simulink model "Sensors_and_actuators_ball_and_plate_2022b"  (R2022b)
settings: Solver=ode1  StartTime=0.0  StopTime=Inf  FixedStep=0.001  RelTol=1e-3
PostLoadFcn:
  | , if any(exist('dsrtsu_mdlpostloadfcn', 'file') ~= 0), dsrtsu_mdlpostloadfcn('Execute', bdroot); end,
InitFcn:
  | , if any(exist('rtifpga_mdlclblib', 'file') ~= 0), rtifpga_mdlclblib('Init', bdroot); end,
values from neighbouring files (symbols this model uses):
  a_y = ((0.1950)-(-0.1950))/(max_py-min_py)    [coordinate_transform.m]    (also in linearmap.m)
  b_x = -0.1950-(a_x*min_px)    [coordinate_transform.m]    (also in linearmap.m)
  b_y = -0.1950-(a_y*min_py)    [coordinate_transform.m]    (also in linearmap.m)
  center = cal1 + ((cal3-cal1)/2)    [coordinate_transform.m]    (also in linearmap.m)
libraries: rtiemclib x6, slpidlib x5, rtiethernetlib x3, rti1202lib_dac_class1 x3
(part 1 of 3)
Description:
  | Standard RTI1202 template.
  | Supported MATLAB version:  R2019b.
settings Model: Tag=RTI1202  DSRTSU_INTERNAL_RTI_VER=570  DSRTSU_INTERNAL_RTI_TYPE=rti1202  RTICANMMDATA=struct('GeneralSetupData',struct('modelroot','C:\Users\20203985\Documents\MATLAB\19_06_2023\simulink','generalsettings',struct('filesettings',struct('destfolder',struct('Name','RTICANMM_FILES','Check',1),'buildfolder',struct('Name','.','Check',1),'AbsDestfolder',struct('Name','C:\Users\20203985\Documents\MATLAB\19_06_2023\simulink\RTICANMM_FILES'),'AbsBuildfolder',struct('Name','C:\Users\20203985\Documents\MATLAB\19_06_2023\simulink'))),'options',struct('addpaths',1,'rmpaths',1,'addtrcexclusion',true,'cannavigator',struct('checkmonitoring',0),'show_usrtrc',0,'use_usrtrc',0),'advanced',struct('options',ones(1,100)),'MPSetup',{{}},'RTI',struct('Type','RTI1202','Ver','7.15','Date','02-Nov-2020'),'modelname','Sensors_and_actuators_ball_and_plate_2022b','block','Sensors_and_actuators_ball_and_plate_2022b'))  DSRTSU_INTERNAL_RTIFPGA=170  Creator=20201603  LastModifiedBy=20203985
settings SolverCC: AlgebraicLoopSolver=TrustRegion
settings DataIOCC: ReturnWorkspaceOutputs=off
settings OptimizationCC: BlockReduction=off  OptimizeBlockIOStorage=off  BufferReuse=off  GlobalBufferReuse=off  ExpressionFolding=off  LocalBlockOutputs=off  OptimizeDataStoreBuffers=off  BusAssignmentInplaceUpdate=off
settings DebuggingCC: ParameterOverflowMsg=none  UnconnectedInputMsg=warning  UnconnectedOutputMsg=warning  UnconnectedLineMsg=warning  PregeneratedLibrarySubsystemCodeDiagnostic=none  ArithmeticOperatorsInVariantConditions=warning
settings HardwareCC: ProdBitPerPointer=32  ProdBitPerSizeT=32  ProdBitPerPtrDiffT=32  ProdLargestAtomicInteger=Integer  ProdEndianess=BigEndian  ProdWordSize=32  ProdLongLongMode=on  ProdHWDeviceType=Custom Processor->Custom  TargetIntDivRoundTo=Zero  TargetEndianess=BigEndian  TargetHWDeviceType=Custom Processor->Custom
settings ModelReferenceCC: EnableRefExpFcnMdlSchedulingChecks=on  EnableParallelModelReferenceBuilds=on  ParallelModelReferenceMATLABWorkerInit=Load Top Model
settings SFSimCC: SimUseLocalCustomCode=off  MATLABDynamicMemAlloc=off  CustomCodeUndefinedFunction=UseInterfaceOnly
settings RTWCC: Description=dSPACE DS1202 Hardware Platform  SystemTargetFile=rti1202.tlc  MakeCommand=make_rti  TemplateMakefile=rti1202.tmf  RTWUseLocalCustomCode=off
settings CodeAppCC: StateflowObjectComments=on
settings STFCustomTargetCC: ParMdlRefBuildCompliant=on  SystemTargetFile=rti1202.tlc
settings GRTTargetCC: TargetLangStandard=C89/C90 (ANSI)  CompOptLevelCompliant=off  ConcurrentExecutionCompliant=off  CombineOutputUpdateFcns=off  MatFileLogging=off  CPPClassGenCompliant=off  UseToolchainInfoCompliant=off
settings ConfigComp: CovMetricSettings=dswe

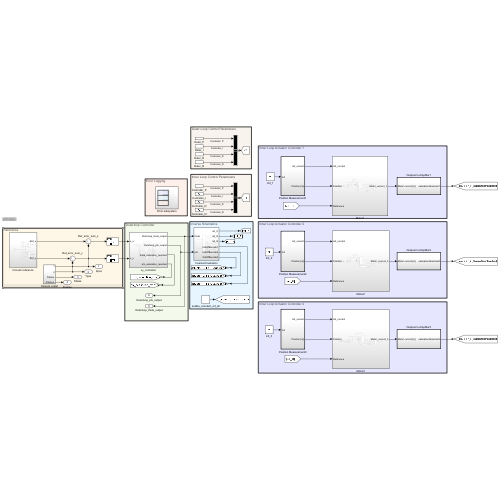
[thumbnail: Simulink's stored preview of the top-level diagram]
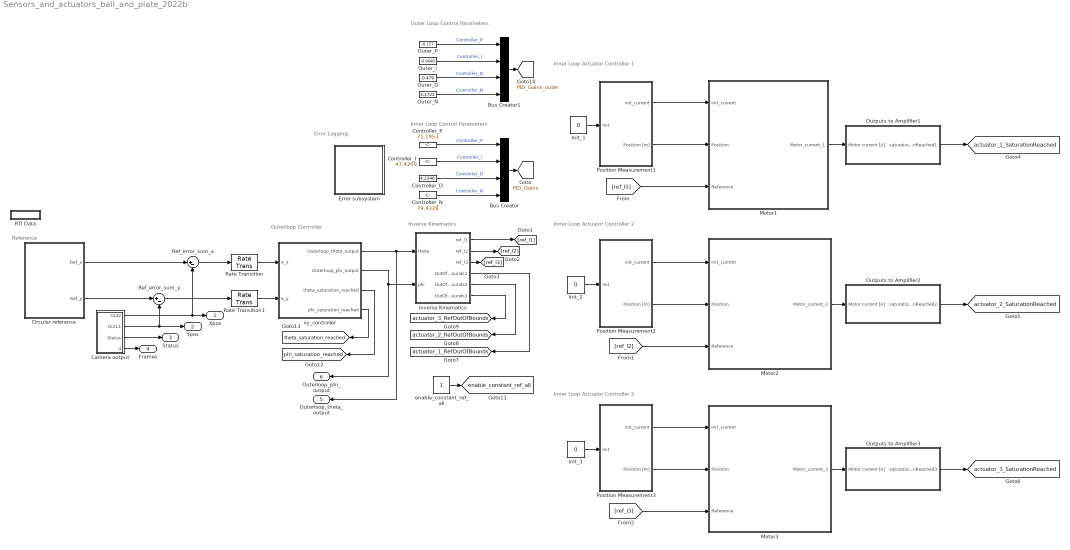
== system Sensors_and_actuators_ball_and_plate_2022b ==
  note: Inner Loop Control Parameters
  note: Error Logging
  note: Inverse Kinematics
  note: Inner Loop Actuator Controller 1
  note: Inner Loop Actuator Controller 2
  note: Inner Loop Actuator Controller 2
  note: Outerloop Controller
  note: Reference
  note: Outer Loop Control Parameters
  Bus Creator : BusCreator  Inputs=4
  Bus Creator1 : BusCreator  Inputs=4
  Camera output : Subsystem
  Circular reference : Subsystem
  Controller_D : Constant  Value=4.2346
  Controller_I : Constant  Value=47.4209
  Controller_N : Constant  Value=79.4328
  Controller_P : Constant  Value=71.1953
  Error subsystem : Subsystem
  Init_1 : Constant  Value=0
  Init_2 : Constant  Value=0
  Inverse Kinematics : Subsystem
  Motor1 : Subsystem
  Motor2 : Subsystem
  Motor3 : Subsystem
  Outer_D : Constant  Value=-0.479
  Outer_I : Constant  Value=-0.0648
  Outer_N : Constant  Value=3.1722
  Outer_P : Constant  Value=-0.157
  Outputs to Amplifier1 : Subsystem  TreatAsAtomicUnit=on
  Outputs to Amplifier2 : Subsystem  TreatAsAtomicUnit=on
  Outputs to Amplifier3 : Subsystem  TreatAsAtomicUnit=on
  Position Measurement1 : Subsystem  TreatAsAtomicUnit=on
  Position Measurement2 : Subsystem  TreatAsAtomicUnit=on
  Position Measurement3 : Subsystem  TreatAsAtomicUnit=on
  RTI Data : Subsystem  Tag=struct('RTIDataServer',struct('RTIDataServerVs','2','RTIModelDescription','struct(''main'',''Sensors_and_actuators_ball_and_plate_2022b'',''sub'','''',''isMp'',0)'))  LoadFcn="if exist('rtidc'), try,  rtidc('DataHostBlockClbLoad', gcbh); catch, disp(['Warning: ''LoadFcn'' for RTI Data block failed: ' lasterr]); end, end,"  mask(RTI_DATA_HOST){}
      mask help:
      | RTI Data Block.
      | This block is used by RTI to store internal model-dependent data.
      | Please keep this block on the root level of the model. Deleting this block will result in data loss.
      |
      | NEVER DELETE OR COPY THIS BLOCK!
      settings: CopyFcn="if exist('rtidc'), try,  rtidc('DataHostBlockClbCopy', gcbh); catch, disp(['Warning: ''CopyFcn'' for RTI Data block failed: ' lasterr]); end, end,"  DeleteFcn="if exist('rtidc'), try,  rtidc('DataHostBlockClbDelete', gcbh); catch, disp(['Warning: ''DeleteFcn'' for RTI Data block failed: ' lasterr]); end, end,"  ModelCloseFcn="if exist('rtidc'), try,  rtidc('DataHostBlockClbModelClose', gcbh); catch, disp(['Warning: ''ModelCloseFcn'' for RTI Data block failed: ' lasterr]); end, end,"  PreSaveFcn="if exist('rtidc'), try,  rtidc('DataHostBlockClbPreSave', gcbh); catch, disp(['Warning: ''PreSaveFcn'' for RTI Data block failed: ' lasterr]); end, end,"  PostSaveFcn="if exist('rtidc'), try,  rtidc('DataHostBlockClbPostSave', gcbh); catch, disp(['Warning: ''PostSaveFcn'' for RTI Data block failed: ' lasterr]); end, end,"  NameChangeFcn="if exist('rtidc'), try,  rtidc('DataHostBlockClbNameChange', gcbh); catch, disp(['Warning: ''NameChangeFcn'' for RTI Data block failed: ' lasterr]); end, end,"
      mask Help:
      | RTI Data Block.
      | This block is used by RTI to store internal model-dependent data.
      | Please keep this block on the root level of the model. Deleting this block will result in data loss.
      | 
      | NEVER DELETE OR COPY THIS BLOCK!
      mask Display:
      | text(0.5, 0.5, 'RTI Data', 'HorizontalAlignment', 'center');
      | plot([1 0]);
  Rate Transition : RateTransition  OutPortSampleTime=0.1
  Rate Transition1 : RateTransition  OutPortSampleTime=0.1
  Ref_error_sum_x : Sum  Inputs=|+-
  Ref_error_sum_y : Sum  Inputs=|+-
  enable_constant_ref_all : Constant
  init_3 : Constant  Value=0
  xy_controller : Subsystem
  "Xpos " : Outport
  "Ypos " : Outport  Port=2
  "Status " : Outport  Port=3
  "Frames " : Outport  Port=4
  Outerloop_theta_output : Outport  Port=5
  Outerloop_phi_output : Outport  Port=6
  tag scope: PID_Gains=global, PID_Gains_outer=global, actuator_1_RefOutOfBounds=global, actuator_1_SaturationReached=global, actuator_2_RefOutOfBounds=global, actuator_2_SaturationReached=global, actuator_3_RefOutOfBounds=global, actuator_3_SaturationReached=global, enable_constant_ref_all=global, phi_saturation_reached=global, theta_saturation_reached=global
  wires:
  Init_1/1 -> Position Measurement1/1(Init)
  init_3/1 -> Position Measurement3/1(Init)
  Controller_P/1 -> Bus Creator/1  "Controller_P"
  Controller_I/1 -> Bus Creator/2  "Controller_I"
  Controller_D/1 -> Bus Creator/3  "Controller_D"
  Controller_N/1 -> Bus Creator/4  "Controller_N"
  Position Measurement1/1(init_current) -> Motor1/1(Init_current)
  Position Measurement1/2(Position [m]) -> Motor1/2(Position)
  Motor1/1(Motor_current_1) -> Outputs to Amplifier1/1(Motor current [A])
  Position Measurement2/1(init_current) -> Motor2/1(Init_current)
  Position Measurement2/2(Position [m]) -> Motor2/2(Position)
  Motor2/1(Motor_current_2) -> Outputs to Amplifier2/1(Motor current [A])
  Position Measurement3/1(init_current) -> Motor3/1(Init_current)
  Position Measurement3/2(Position [m]) -> Motor3/2(Position)
  Motor3/1(Motor_current_3) -> Outputs to Amplifier3/1(Motor current [A])
  Circular reference/1(Ref_x) -> Ref_error_sum_x/1
  Circular reference/2(Ref_y) -> Ref_error_sum_y/1
  Camera output/1(Out2) -> "Xpos "/1, Ref_error_sum_x/2
  Camera output/2(Out11) -> "Ypos "/1, Ref_error_sum_y/2
  Camera output/3("Status ") -> "Status "/1
  Camera output/4("Frames ") -> "Frames "/1
  Ref_error_sum_x/1 -> Rate Transition/1
  Ref_error_sum_y/1 -> Rate Transition1/1
  Init_2/1 -> Position Measurement2/1(Init)
  Inverse Kinematics/2(ref_l2) -> [ref_l2]
  Inverse Kinematics/3(ref_l3) -> [ref_l3]
  Inverse Kinematics/1(ref_l1) -> [ref_l1]
  [ref_l1] -> Motor1/3(Reference)
  [ref_l2] -> Motor2/3(Reference)
  [ref_l3] -> Motor3/3(Reference)
  xy_controller/1(Outerloop_theta_output) -> Outerloop_theta_output/1, Inverse Kinematics/1(theta)
  xy_controller/2(Outerloop_phi_output) -> Outerloop_phi_output/1, Inverse Kinematics/2(phi)
  Bus Creator/1 -> [PID_Gains]
  Inverse Kinematics/4(OutOfBounds1) -> [actuator_1_RefOutOfBounds]
  Inverse Kinematics/5(OutOfBounds2) -> [actuator_2_RefOutOfBounds]
  Inverse Kinematics/6(OutOfBounds3) -> [actuator_3_RefOutOfBounds]
  Outputs to Amplifier1/1(saturationReached1) -> [actuator_1_SaturationReached]
  Outputs to Amplifier2/1(saturationReached2) -> [actuator_2_SaturationReached]
  Outputs to Amplifier3/1(saturationReached3) -> [actuator_3_SaturationReached]
  Outer_N/1 -> Bus Creator1/4  "Controller_N"
  Bus Creator1/1 -> [PID_Gains_outer]
  Outer_D/1 -> Bus Creator1/3  "Controller_D"
  Outer_P/1 -> Bus Creator1/1  "Controller_P"
  Outer_I/1 -> Bus Creator1/2  "Controller_I"
  enable_constant_ref_all/1 -> [enable_constant_ref_all]
  xy_controller/4(phi_saturation_reached) -> [theta_saturation_reached]
  xy_controller/3(theta_saturation_reached) -> [phi_saturation_reached]
  Rate Transition/1 -> xy_controller/1(e_x)
  Rate Transition1/1 -> xy_controller/2(e_y)

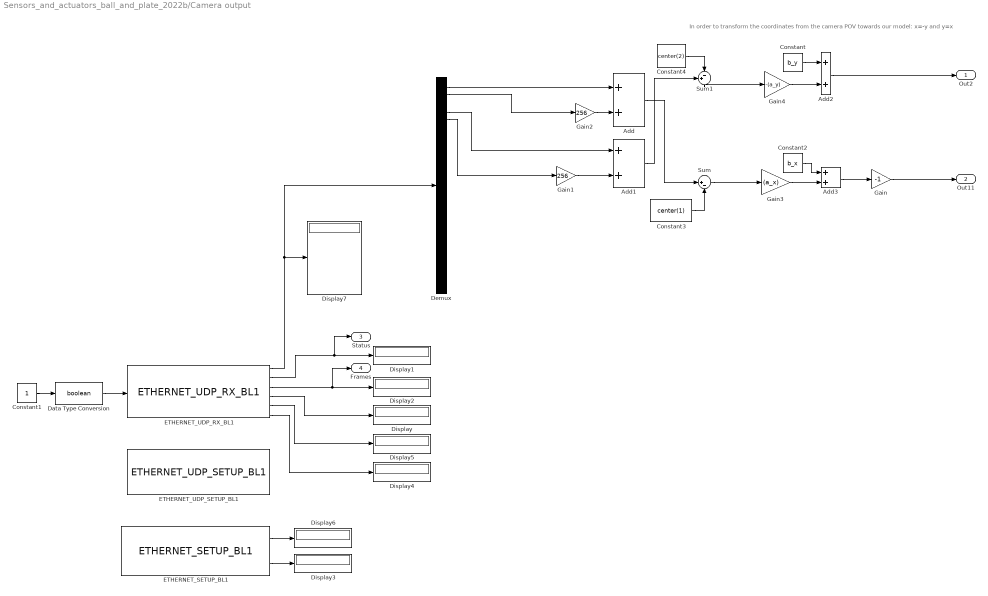
== system Sensors_and_actuators_ball_and_plate_2022b/Camera output ==
  note: In order to transform the coordinates from the camera POV towards our model: x=-y and y=x
  Add : Sum  AccumDataTypeStr=uint16
  Add1 : Sum
  Add2 : Sum
  Add3 : Sum
  Constant : Constant  Value=b_y
  Constant1 : Constant
  Constant2 : Constant  Value=b_x
  Constant3 : Constant  Value=center(1)
  Constant4 : Constant  Value=center(2)
  Data Type Conversion : DataTypeConversion  OutDataTypeStr=boolean  SaturateOnIntegerOverflow=off  RndMeth=Floor
  Demux : Demux  Outputs=32
  Display{,1..7} (8 alike) : Display
      Display7 settings: Format=decimal (Stored Integer)
  ETHERNET_SETUP_BL1 : rtiethernetlib/ETHERNET_SETUP_BL1  DSProperties=struct('RTI',struct('Version',uint32(2),'BlockType',struct('isSLSource',uint8(0),'isSLSink',uint8(0),'isHWSource',uint8(0),'isHWSink',uint8(0),'isSetup',uint8(1),'isInline',uint8(1),'isNonInline',uint8(0),'isInterrupt',uint8(0),'isChannelwise',uint8(0)),'IOBoardType','DSETHERNET','UnitType','ETHERNET','Identifier','SETUP','DialogType','ML','BlockSet','RTIETHERNET','SlaveProcessor','NONE'))  RTIBlockInterface=struct('OutputPortsWidth',int32([3 1 1 4]),'OutputPortsActive',[1 0 0 1],'OutputPortsName',{{['Link Status'],['Watchdog Status'],['DHCP Status'],['Local IP']}},'OutputPortsDataType',{{'SS_UINT32','SS_UINT32','SS_UINT32','SS_UINT8'}},'InitLevel',3,'IconTransparency','on','BlockDisplay',{{['Ethernet Setup\n\nLocal IP: 192.168.141.7'],'left'}},'DialogFcn','rtiethernetsetupgui','BlockName',struct('Token',{{'ETHERNET_SETUP_BL1'}}))  RTIBlockParameters=struct('DHCPserverMode',{{0,'OFF',[0 1]}},'LocalIpNum1',{{'192','OFF',[0 255]}},'LocalIpNum2',{{'168','OFF',[0 255]}},'LocalIpNum3',{{'141','OFF',[0 255]}},'LocalIpNum4',{{'7','OFF',[0 255]}},'SubnetMaskNum1',{{'255','OFF',[0 255]}},'SubnetMaskNum2',{{'255','OFF',[0 255]}},'SubnetMaskNum3',{{'255','OFF',[0 255]}},'SubnetMaskNum4',{{'0','OFF',[0 255]}},'GatewayNum1',{{'0','OFF',[0 255]}},'GatewayNum2',{{'0','OFF',[0 255]}},'GatewayNum3',{{'0','OFF',[0 255]}},'GatewayNum4',{{'0','OFF',[0 255]}},'LinkStatusOutPortMode',{{1,'OFF',[0 1]}},'NumOfEthConnectors',{{3,'ON',[1 16]}},'WatchdogStatusOutPortMode',{{0,'OFF',[0 1]}},'LocalIpOutPortMode',{{1,'OFF',[0 1]}},'IpAndSubmaskCheck',{{int32(1),'OFF',[0 1]}},'TLCFileName',{{'rtiethernetsetup','OFF',[]}})  RTISFcnParameters=struct('DHCPserverMode','int32','LocalIpNum1','uint8','LocalIpNum2','uint8','LocalIpNum3','uint8','LocalIpNum4','uint8','SubnetMaskNum1','uint8','SubnetMaskNum2','uint8','SubnetMaskNum3','uint8','SubnetMaskNum4','uint8','GatewayNum1','uint8','GatewayNum2','uint8','GatewayNum3','uint8','GatewayNum4','uint8','LinkStatusOutPortMode','int32','NumOfEthConnectors','int32','WatchdogStatusOutPortMode','int32','LocalIpOutPortMode','int32','TLCFileName','char')  RTIBlockParaDefault=struct('DHCPserverMode',0,'LocalIpNum1',192,'LocalIpNum2',168,'LocalIpNum3',140,'LocalIpNum4',6,'SubnetMaskNum1',255,'SubnetMaskNum2',255,'SubnetMaskNum3',255,'SubnetMaskNum4',0,'GatewayNum1',0,'GatewayNum2',0,'GatewayNum3',0,'GatewayNum4',0,'LinkStatusOutPortMode',1,'NumOfEthConnectors',3,'WatchdogStatusOutPortMode',0,'LocalIpOutPortMode',0,'IpAndSubmaskCheck',1,'TLCFileName','rtiethernetsetup')
      settings: SourceProductName=dSPACE RTI Ethernet Blockset
  ETHERNET_UDP_RX_BL1 : rtiethernetlib/ETHERNET_UDP_RX_BL1  DSProperties=struct('RTI',struct('Version',uint32(1),'BlockType',struct('isSLSource',uint8(1),'isSLSink',uint8(1),'isHWSource',uint8(0),'isHWSink',uint8(1),'isSetup',uint8(0),'isInline',uint8(1),'isNonInline',uint8(0),'isInterrupt',uint8(0),'isChannelwise',uint8(0)),'IOBoardType','DSETHERNET','UnitType','UDP','Identifier','RXUDP','DialogType','ML','BlockSet','RTIETHERNET','SlaveProcessor','NONE'))  RTIBlockInterface=struct('OutputPortsWidth',int32([32 1 1 1 4 1]),'OutputPortsActive',[1 1 1 1 1 1],'OutputPortsName',{{'Data','Status',['Received Frames'],['Received Bytes'],['Remote IP'],['Remote Port']}},'OutputPortsDataType',{{'SS_UINT8','SS_UINT32','SS_DOUBLE','SS_UINT32','SS_UINT8','SS_UINT16'}},'InputPortsWidth',int32(1),'InputPortsActive',1,'InputPortsName',{{'Enable'}},'InputPortsDataType',{{'SS_BOOLEAN'}},'RWork',{{{'RECEIVED_FRAMES',uint32(1)}}},'InitLevel',3,'IconTransparency','on','BlockDisplay',{{['Ethernet UDP/IP\nRX\n\nSocket ID: 0'],'center'}},'DialogFcn','rtiethernetrxudpgui','BlockName',struct('Token',{{'ETHERNET_UDP_RX_BL1'}}))  RTIBlockParameters=struct('SocketIdIndex',{{2,'OFF',[1 2]}},'SocketId',{{0,'OFF',[-1 inf]}},'RemoteIp',{{['<NOT AVAILABLE>'],'OFF',[]}},'RemotePort',{{['<NOT AVAILABLE>'],'OFF',[]}},'LocalPort',{{49001,'OFF',[]}},'FrameSize',{{'32','OFF',[1 65507]}},'EnableVariableFrameSize',{{1,'OFF',[0 1]}},'VariableFrameSizeMode',{{1,'OFF',[1 2]}},'InterruptMode',{{0,'OFF',[0 1]}},'RemoteIpOutPortMode',{{1,'OFF',[0 1]}},'RemotePortOutPortMode',{{1,'OFF',[0 1]}},'TLCFileName',{{'rtiethernetrxudp','OFF',[]}})  RTISFcnParameters=struct('SocketIdIndex','int32','SocketId','double','FrameSize','uint16','EnableVariableFrameSize','int32','VariableFrameSizeMode','int32','InterruptMode','int32','RemoteIpOutPortMode','int32','RemotePortOutPortMode','int32','TLCFileName','char')  RTIBlockParaDefault=struct('SocketIdIndex',1,'SocketId',-1,'RemoteIp',['<NOT AVAILABLE>'],'RemotePort',['<NOT AVAILABLE>'],'LocalPort',['<NOT AVAILABLE>'],'FrameSize',1024,'EnableVariableFrameSize',0,'VariableFrameSizeMode',1,'InterruptMode',0,'RemoteIpOutPortMode',0,'RemotePortOutPortMode',0,'TLCFileName','rtiethernetrxudp')
      settings: SourceProductName=dSPACE RTI Ethernet Blockset
  ETHERNET_UDP_SETUP_BL1 : rtiethernetlib/ETHERNET_UDP_SETUP_BL1  DSProperties=struct('RTI',struct('Version',uint32(2),'BlockType',struct('isSLSource',uint8(1),'isSLSink',uint8(1),'isHWSource',uint8(0),'isHWSink',uint8(0),'isSetup',uint8(0),'isInline',uint8(1),'isNonInline',uint8(0),'isInterrupt',uint8(0),'isChannelwise',uint8(0)),'IOBoardType','DSETHERNET','UnitType','UDP','Identifier','SETUPUDP','DialogType','ML','BlockSet','RTIETHERNET','SlaveProcessor','NONE'))  RTIBlockInterface=struct('OutputPortsWidth',int32(2),'OutputPortsActive',0,'OutputPortsName',{{['RX Dropped Frames']}},'OutputPortsDataType',{{'SS_DOUBLE'}},'InputPortsWidth',int32([4 1]),'InputPortsActive',int32([0 0]),'InputPortsName',{{['RX Remote IP Filter'],['RX Remote Port Filter']}},'InputPortsDataType',{{'SS_UINT8','SS_UINT16'}},'RWork',{{{'RX_DROPPED_FRAMES',uint32(2)}}},'InitLevel',3,'IconTransparency','on','BlockDisplay',{{['Ethernet UDP/IP\nSetup\n\nSocket ID: 0'],'center'}},'DialogFcn','rtiethernetsetupudpgui','BlockName',struct('Token',{{'ETHERNET_UDP_SETUP_BL1'}}))  RTIBlockParameters=struct('SocketId',{{0,'OFF',[]}},'EnableSocketBind',{{1,'OFF',[0 1]}},'AcceptAnyRxRemoteIp',{{1,'OFF',[0 1]}},'RxRemoteIpNum1',{{'131','OFF',[0 255]}},'RxRemoteIpNum2',{{'155','OFF',[0 255]}},'RxRemoteIpNum3',{{'33','OFF',[0 255]}},'RxRemoteIpNum4',{{'44','OFF',[0 255]}},'EnableDynamicRxRemoteIpFilter',{{0,'OFF',[0 1]}},'AcceptAnyRxRemotePort',{{1,'OFF',[0 1]}},'RxRemotePort',{{'57272','OFF',[1 65535]}},'EnableDynamicRxRemotePortFilter',{{0,'OFF',[0 1]}},'TxRemoteIpNum1',{{'131','OFF',[0 255]}},'TxRemoteIpNum2',{{'155','OFF',[0 255]}},'TxRemoteIpNum3',{{'33','OFF',[0 255]}},'TxRemoteIpNum4',{{'44','OFF',[0 255]}},'TxRemotePort',{{'49002','OFF',[1 65535]}},'SpecifyLocalPort',{{1,'OFF',[0 1]}},'LocalPort',{{'49001','OFF',[1 65535]}},'InterruptMode',{{0,'OFF',[0 1]}},'RxDroppedFramesOutPortMode',{{0,'OFF',[0 1]}},'RemoteIpNumCheck',{{0,'OFF',[0 1]}},'RemotePortCheck',{{0,'OFF',[0 1]}},'LocalPortCheck',{{1,'OFF',[0 1]}},'DHCPserverModeEnabled',{{0,'OFF',[0 1]}},'TLCFileName',{{'rtiethernetsetupudp','OFF',[]}})  RTISFcnParameters=struct('SocketId','double','EnableSocketBind','int32','AcceptAnyRxRemoteIp','int32','RxRemoteIpNum1','uint8','RxRemoteIpNum2','uint8','RxRemoteIpNum3','uint8','RxRemoteIpNum4','uint8','EnableDynamicRxRemoteIpFilter','int32','AcceptAnyRxRemotePort','int32','RxRemotePort','uint16','EnableDynamicRxRemotePortFilter','int32','TxRemoteIpNum1','uint8','TxRemoteIpNum2','uint8','TxRemoteIpNum3','uint8','TxRemoteIpNum4','uint8','TxRemotePort','uint16','SpecifyLocalPort','int32','LocalPort','uint16','InterruptMode','int32','RxDroppedFramesOutPortMode','int32','DHCPserverModeEnabled','int32','TLCFileName','char')  RTIBlockParaDefault=struct('SocketId',-1,'EnableSocketBind',1,'AcceptAnyRxRemoteIp',1,'RxRemoteIpNum1',0,'RxRemoteIpNum2',0,'RxRemoteIpNum3',0,'RxRemoteIpNum4',0,'EnableDynamicRxRemoteIpFilter',0,'AcceptAnyRxRemotePort',1,'RxRemotePort',49002,'EnableDynamicRxRemotePortFilter',0,'TxRemoteIpNum1',0,'TxRemoteIpNum2',0,'TxRemoteIpNum3',0,'TxRemoteIpNum4',0,'TxRemotePort',49002,'SpecifyLocalPort',0,'LocalPort',49001,'InterruptMode',0,'RxDroppedFramesOutPortMode',0,'RemoteIpNumCheck',0,'RemotePortCheck',0,'LocalPortCheck',0,'DHCPserverModeEnabled',0,'TLCFileName','rtiethernetsetupudp')
      settings: SourceProductName=dSPACE RTI Ethernet Blockset
  Gain : Gain  Gain=-1
  Gain1 : Gain  Gain=256  OutDataTypeStr=uint16
  Gain2 : Gain  Gain=256  OutDataTypeStr=uint16
  Gain3 : Gain  Gain=(a_x)
  Gain4 : Gain  Gain=-(a_y)
  Sum : Sum  Inputs=|+-
  Sum1 : Sum  Inputs=+-|
  Out2 : Outport
  Out11 : Outport  Port=2
  "Status " : Outport  Port=3
  "Frames " : Outport  Port=4
  wires:
  Demux/5 -> Add1/1
  Gain2/1 -> Add/2
  Demux/6 -> Gain1/1
  Demux/1 -> Add/1
  ETHERNET_UDP_RX_BL1/6 -> Display4/1
  ETHERNET_UDP_RX_BL1/1 -> Demux/1, Display7/1
  ETHERNET_UDP_RX_BL1/2 -> "Status "/1, Display1/1
  Data Type Conversion/1 -> ETHERNET_UDP_RX_BL1/1
  Demux/2 -> Gain2/1
  Gain1/1 -> Add1/2
  ETHERNET_SETUP_BL1/1 -> Display6/1
  ETHERNET_UDP_RX_BL1/3 -> "Frames "/1, Display2/1
  Constant1/1 -> Data Type Conversion/1
  ETHERNET_UDP_RX_BL1/4 -> Display/1
  ETHERNET_UDP_RX_BL1/5 -> Display5/1
  ETHERNET_SETUP_BL1/2 -> Display3/1
  Constant/1 -> Add2/1
  Gain3/1 -> Add3/2
  Constant2/1 -> Add3/1
  Add3/1 -> Gain/1
  Gain4/1 -> Add2/2
  Add/1 -> Sum/1
  Constant3/1 -> Sum/2
  Sum/1 -> Gain3/1
  Add1/1 -> Sum1/1
  Constant4/1 -> Sum1/2
  Sum1/1 -> Gain4/1
  Add2/1 -> Out2/1
  Gain/1 -> Out11/1

== system Sensors_and_actuators_ball_and_plate_2022b/Circular reference ==
  Sine Wave : Sin  Amplitude=0.1  Frequency=0.25*2*pi  Phase=pi/2  SampleTime=0
  Sine Wave1 : Sin  Amplitude=0.1  Frequency=0.25*2*pi  SampleTime=0
  Switch : Switch  Threshold=0.5  SaturateOnIntegerOverflow=off  InputSameDT=off
  Switch1 : Switch  Threshold=0.5  SaturateOnIntegerOverflow=off  InputSameDT=off
  circle_reference_on : Constant  Value=0
  ref_x_constant : Constant  Value=0
  ref_y_constant : Constant  Value=0
  Ref_x : Outport
  Ref_y : Outport  Port=2
  wires:
  Switch1/1 -> Ref_y/1
  Switch/1 -> Ref_x/1
  circle_reference_on/1 -> Switch1/2, Switch/2
  Sine Wave/1 -> Switch/1
  ref_x_constant/1 -> Switch/3
  ref_y_constant/1 -> Switch1/3
  Sine Wave1/1 -> Switch1/1

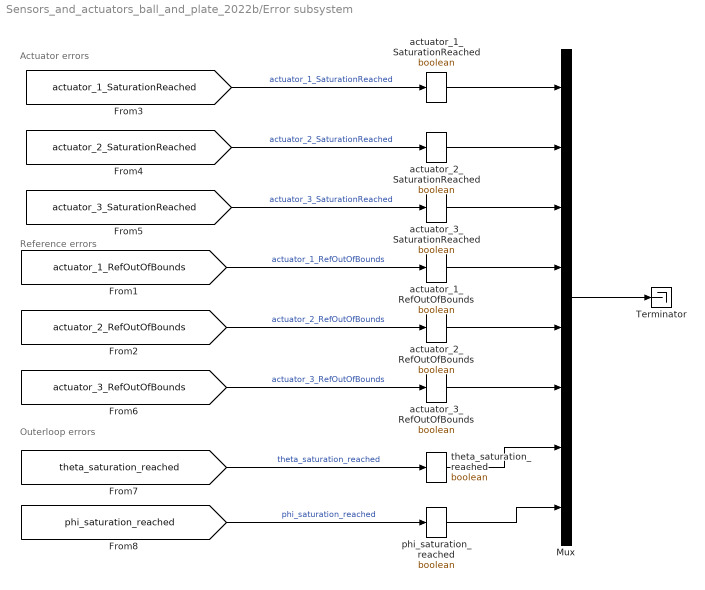
== system Sensors_and_actuators_ball_and_plate_2022b/Error subsystem ==
  note: Actuator errors
  note: Reference errors
  note: Outerloop errors
  Mux : Mux  Inputs=8
  Terminator : Terminator
  actuator_1_RefOutOfBounds : DataTypeConversion  OutDataTypeStr=boolean  SaturateOnIntegerOverflow=off  RndMeth=Floor
  actuator_1_SaturationReached : DataTypeConversion  OutDataTypeStr=boolean  SaturateOnIntegerOverflow=off  RndMeth=Floor
  actuator_2_RefOutOfBounds : DataTypeConversion  OutDataTypeStr=boolean  SaturateOnIntegerOverflow=off  RndMeth=Floor
  actuator_2_SaturationReached : DataTypeConversion  OutDataTypeStr=boolean  SaturateOnIntegerOverflow=off  RndMeth=Floor
  actuator_3_RefOutOfBounds : DataTypeConversion  OutDataTypeStr=boolean  SaturateOnIntegerOverflow=off  RndMeth=Floor
  actuator_3_SaturationReached : DataTypeConversion  OutDataTypeStr=boolean  SaturateOnIntegerOverflow=off  RndMeth=Floor
  phi_saturation_reached : DataTypeConversion  OutDataTypeStr=boolean  SaturateOnIntegerOverflow=off  RndMeth=Floor
  theta_saturation_reached : DataTypeConversion  OutDataTypeStr=boolean  SaturateOnIntegerOverflow=off  RndMeth=Floor
  wires:
  [actuator_2_SaturationReached] -> actuator_2_SaturationReached/1  "actuator_2_SaturationReached"
  [actuator_1_SaturationReached] -> actuator_1_SaturationReached/1  "actuator_1_SaturationReached"
  [actuator_3_SaturationReached] -> actuator_3_SaturationReached/1  "actuator_3_SaturationReached"
  Mux/1 -> Terminator/1
  [actuator_1_RefOutOfBounds] -> actuator_1_RefOutOfBounds/1  "actuator_1_RefOutOfBounds"
  [actuator_2_RefOutOfBounds] -> actuator_2_RefOutOfBounds/1  "actuator_2_RefOutOfBounds"
  [actuator_3_RefOutOfBounds] -> actuator_3_RefOutOfBounds/1  "actuator_3_RefOutOfBounds"
  actuator_1_SaturationReached/1 -> Mux/1
  actuator_2_SaturationReached/1 -> Mux/2
  actuator_3_SaturationReached/1 -> Mux/3
  actuator_1_RefOutOfBounds/1 -> Mux/4
  actuator_2_RefOutOfBounds/1 -> Mux/5
  actuator_3_RefOutOfBounds/1 -> Mux/6
  [theta_saturation_reached] -> theta_saturation_reached/1  "theta_saturation_reached"
  [phi_saturation_reached] -> phi_saturation_reached/1  "phi_saturation_reached"
  theta_saturation_reached/1 -> Mux/7
  phi_saturation_reached/1 -> Mux/8

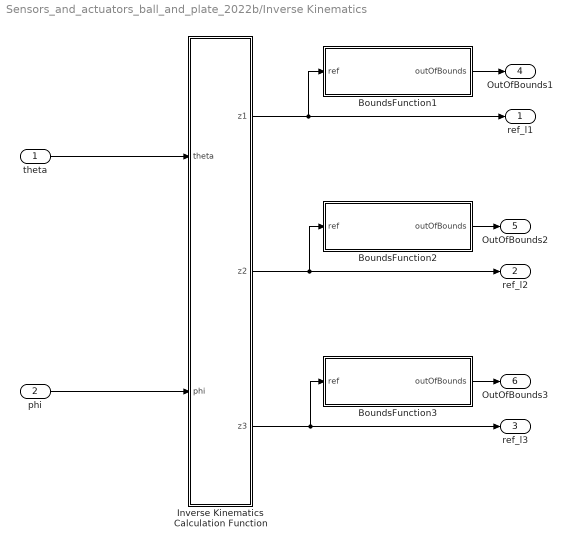
== system Sensors_and_actuators_ball_and_plate_2022b/Inverse Kinematics ==
  theta : Inport
  phi : Inport  Port=2
  BoundsFunction1 : MATLAB Function  TreatAsAtomicUnit=on
  BoundsFunction2 : MATLAB Function  TreatAsAtomicUnit=on
  BoundsFunction3 : MATLAB Function  TreatAsAtomicUnit=on
  Inverse Kinematics Calculation Function : MATLAB Function  TreatAsAtomicUnit=on
  ref_l1 : Outport
  ref_l2 : Outport  Port=2
  ref_l3 : Outport  Port=3
  OutOfBounds1 : Outport  Port=4
  OutOfBounds2 : Outport  Port=5
  OutOfBounds3 : Outport  Port=6
  wires:
  Inverse Kinematics Calculation Function/2(z2) -> BoundsFunction2/1(ref), ref_l2/1
  Inverse Kinematics Calculation Function/3(z3) -> BoundsFunction3/1(ref), ref_l3/1
  BoundsFunction1/1(outOfBounds) -> OutOfBounds1/1
  Inverse Kinematics Calculation Function/1(z1) -> BoundsFunction1/1(ref), ref_l1/1
  BoundsFunction2/1(outOfBounds) -> OutOfBounds2/1
  BoundsFunction3/1(outOfBounds) -> OutOfBounds3/1
  phi/1 -> Inverse Kinematics Calculation Function/2(phi)
  theta/1 -> Inverse Kinematics Calculation Function/1(theta)

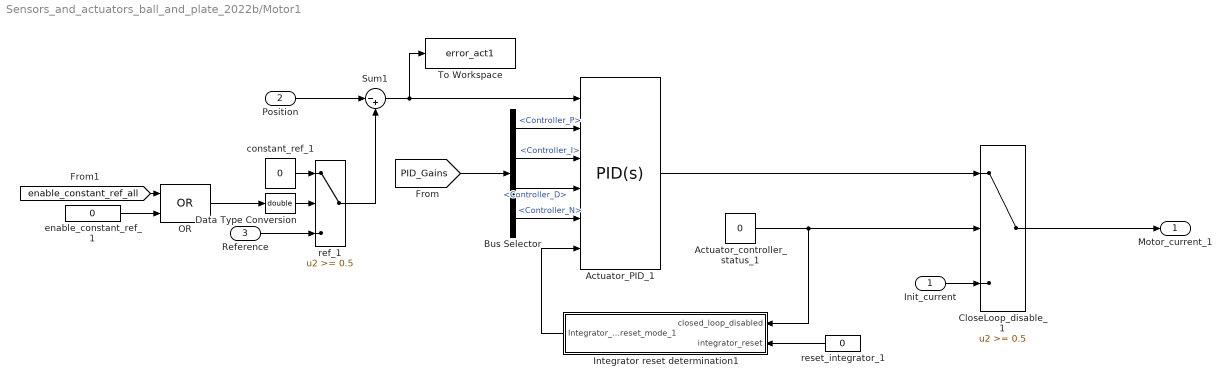
== system Sensors_and_actuators_ball_and_plate_2022b/Motor1 ==
  Init_current : Inport
  Position : Inport  Port=2
  Reference : Inport  Port=3
  Actuator_PID_1 : slpidlib/PID Controller  Controller=PID  Form=Parallel  TimeDomain=Continuous-time  UseExternalTs=off  SampleTime=-1  IntegratorMethod=Forward Euler  FilterMethod=Forward Euler  ControllerParametersSource=external  P=50  I=0  UseKiTs=off  D=0  N=100  UseFilter=on  TunerSelectOption=Transfer Function Based (PID Tuner App)  InitialConditionSource=internal  InitialConditionForIntegrator=0  InitialConditionForFilter=0  DifferentiatorICPrevScaledInput=0  ExternalReset=level  TrackingMode=off  Kt=1  LimitOutput=on  SatLimitsSource=internal  UpperSaturationLimit=3  LowerSaturationLimit=-3  LinearizeAsGain=on  AntiWindupMode=none  Kb=1  LimitIntegrator=off  UpperIntegratorSaturationLimit=inf  LowerIntegratorSaturationLimit=-inf  POutMin=[]  POutMax=[]  IOutMin=[]  IOutMax=[]  DOutMin=[]  DOutMax=[]  NOutMin=[]  NOutMax=[]  SumOutMin=[]  SumOutMax=[]  SaturationOutMin=[]  SaturationOutMax=[]  PParamMin=[]  PParamMax=[]  IParamMin=[]  IParamMax=[]  DParamMin=[]  DParamMax=[]  NParamMin=[]  NParamMax=[]  KbParamMin=[]  KbParamMax=[]  KtParamMin=[]  KtParamMax=[]  KbOutMin=[]  KbOutMax=[]  KtOutMin=[]  KtOutMax=[]  IntegratorOutMin=[]  IntegratorOutMax=[]  FilterOutMin=[]  FilterOutMax=[]  SumI1OutMin=[]  SumI1OutMax=[]  SumI2OutMin=[]  SumI2OutMax=[]  SumI3OutMin=[]  SumI3OutMax=[]  SumI4OutMin=[]  SumI4OutMax=[]  SumDOutMin=[]  SumDOutMax=[]  DifferentiatorOutMin=[]  DifferentiatorOutMax=[]  FilterDiffOutCoefMin=[]  FilterDiffOutCoefMax=[]  ReciprocalOutMin=[]  ReciprocalOutMax=[]  SumDenOutMin=[]  SumDenOutMax=[]  SumNumOutMin=[]  SumNumOutMax=[]  DivideOutMin=[]  DivideOutMax=[]  UdiffTsProdOutMin=[]  UdiffTsProdOutMax=[]  NTsProdOutMin=[]  NTsProdOutMax=[]  UintegralTsProdOutMin=[]  UintegralTsProdOutMax=[]  UngainTsProdOutMin=[]  UngainTsProdOutMax=[]  ClampingZeroOutDataTypeStr=Inherit: Inherit via back propagation  ClampingZeroOutMin=[]  ClampingZeroOutMax=[]  FilterDenConstantOutDataTypeStr=Inherit: Inherit via back propagation  FilterDenConstantOutMin=[]  FilterDenConstantOutMax=[]  PCopyOutDataTypeStr=Inherit: Inherit via back propagation  PCopyOutMin=[]  PCopyOutMax=[]  NCopyOutDataTypeStr=Inherit: Inherit via back propagation  NCopyOutMin=[]  NCopyOutMax=[]  IntegratorContinuousStateAttributes=''  IntegratorStateMustResolveToSignalObject=off  IntegratorRTWStateStorageClass=Auto  FilterContinuousStateAttributes=''  FilterStateMustResolveToSignalObject=off  FilterRTWStateStorageClass=Auto  ParallelPVariant=ExternalParameters  IdealPVariant=Disabled  IVariant=ExternalParameters  DVariant=ExternalParameters  IntegratorVariant=Continuous  SatVariant=Enabled  AWVariant=Passthrough  PCopyVariant=Disabled  TRVariant=Disabled  FdbkBlocksVariant=Forward  IdealPFdbkVariant=Disabled  SatFdbkVariant=Disabled  DerivativeFilterVariant=ContFilter  NVariant=ExternalParameters  NCopyVariant=Disabled  FilterICVariant=InternalICsFilter  IntegratorICVariant=InternalICs  ExternalResetVariant=ExternalReset  TRSumVariant=Passthrough  SumFdbkVariant=Disabled  SumVariant=Sum_PID  TsampFilterVariant=InternalTs  TsampNgainVariant=Passthrough  TsampIntegralVariant=Passthrough  ExternalSaturationOutDataTypeStr=Inherit: Same as second input
  Actuator_controller_status_1 : Constant  Value=0
  Bus Selector : BusSelector  OutputSignals=Controller_P,Controller_I,Controller_D,Controller_N
  CloseLoop_disable_1 : Switch  Threshold=0.5  SaturateOnIntegerOverflow=off  InputSameDT=off
  Data Type Conversion : DataTypeConversion  OutDataTypeStr=double  SaturateOnIntegerOverflow=off  RndMeth=Floor
  Integrator reset determination1 : MATLAB Function  TreatAsAtomicUnit=on
  OR : Logic  Operator=OR  IconShape=distinctive  AllPortsSameDT=off  OutDataTypeStr=boolean
  Sum1 : Sum  Inputs=|-+  SaturateOnIntegerOverflow=on
  To Workspace : ToWorkspace  VariableName=error_act1  SampleTime=-1
  constant_ref_1 : Constant  Value=0
  enable_constant_ref_1 : Constant  Value=0
  ref_1 : Switch  Threshold=0.5  SaturateOnIntegerOverflow=off  InputSameDT=off
  reset_integrator_1 : Constant  Value=0
  Motor_current_1 : Outport
  wires:
  Position/1 -> Sum1/1
  ref_1/1 -> Sum1/2
  Bus Selector/2 -> Actuator_PID_1/3  "<Controller_I>"
  constant_ref_1/1 -> ref_1/1
  [PID_Gains] -> Bus Selector/1
  Bus Selector/1 -> Actuator_PID_1/2  "<Controller_P>"
  Bus Selector/3 -> Actuator_PID_1/4  "<Controller_D>"
  Bus Selector/4 -> Actuator_PID_1/5  "<Controller_N>"
  OR/1 -> Data Type Conversion/1
  Sum1/1 -> To Workspace/1, Actuator_PID_1/1
  Init_current/1 -> CloseLoop_disable_1/3
  Reference/1 -> ref_1/3
  reset_integrator_1/1 -> Integrator reset determination1/2(integrator_reset)
  Actuator_PID_1/1 -> CloseLoop_disable_1/1
  CloseLoop_disable_1/1 -> Motor_current_1/1
  Actuator_controller_status_1/1 -> Integrator reset determination1/1(closed_loop_disabled), CloseLoop_disable_1/2
  Integrator reset determination1/1(Integrator_reset_mode_1) -> Actuator_PID_1/6
  [enable_constant_ref_all] -> OR/1
  enable_constant_ref_1/1 -> OR/2
  Data Type Conversion/1 -> ref_1/2

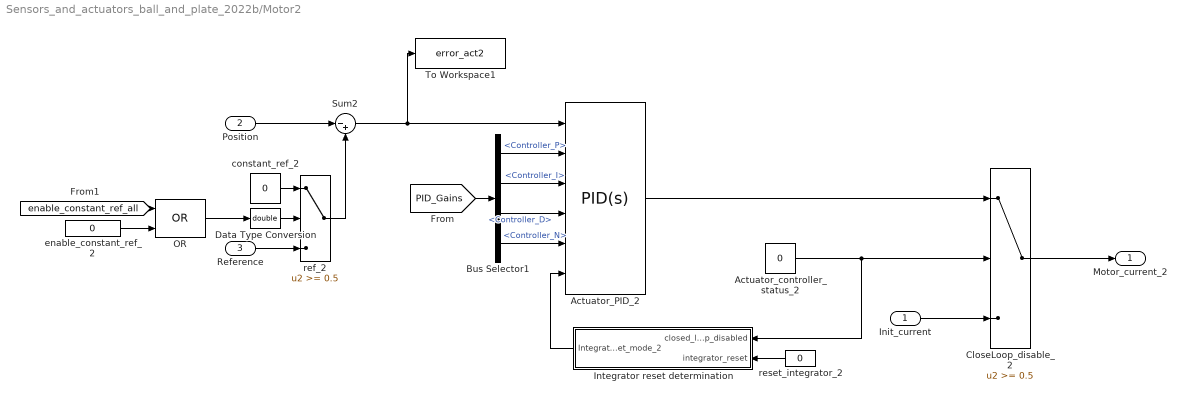
== system Sensors_and_actuators_ball_and_plate_2022b/Motor2 ==
  Init_current : Inport
  Position : Inport  Port=2
  Reference : Inport  Port=3
  Actuator_PID_2 : slpidlib/PID Controller  Controller=PID  Form=Parallel  TimeDomain=Continuous-time  UseExternalTs=off  SampleTime=-1  IntegratorMethod=Forward Euler  FilterMethod=Forward Euler  ControllerParametersSource=external  P=50  I=0  UseKiTs=off  D=0  N=100  UseFilter=on  TunerSelectOption=Transfer Function Based (PID Tuner App)  InitialConditionSource=internal  InitialConditionForIntegrator=0  InitialConditionForFilter=0  DifferentiatorICPrevScaledInput=0  ExternalReset=level  TrackingMode=off  Kt=1  LimitOutput=on  SatLimitsSource=internal  UpperSaturationLimit=3  LowerSaturationLimit=-3  LinearizeAsGain=on  AntiWindupMode=none  Kb=1  LimitIntegrator=off  UpperIntegratorSaturationLimit=inf  LowerIntegratorSaturationLimit=-inf  POutMin=[]  POutMax=[]  IOutMin=[]  IOutMax=[]  DOutMin=[]  DOutMax=[]  NOutMin=[]  NOutMax=[]  SumOutMin=[]  SumOutMax=[]  SaturationOutMin=[]  SaturationOutMax=[]  PParamMin=[]  PParamMax=[]  IParamMin=[]  IParamMax=[]  DParamMin=[]  DParamMax=[]  NParamMin=[]  NParamMax=[]  KbParamMin=[]  KbParamMax=[]  KtParamMin=[]  KtParamMax=[]  KbOutMin=[]  KbOutMax=[]  KtOutMin=[]  KtOutMax=[]  IntegratorOutMin=[]  IntegratorOutMax=[]  FilterOutMin=[]  FilterOutMax=[]  SumI1OutMin=[]  SumI1OutMax=[]  SumI2OutMin=[]  SumI2OutMax=[]  SumI3OutMin=[]  SumI3OutMax=[]  SumI4OutMin=[]  SumI4OutMax=[]  SumDOutMin=[]  SumDOutMax=[]  DifferentiatorOutMin=[]  DifferentiatorOutMax=[]  FilterDiffOutCoefMin=[]  FilterDiffOutCoefMax=[]  ReciprocalOutMin=[]  ReciprocalOutMax=[]  SumDenOutMin=[]  SumDenOutMax=[]  SumNumOutMin=[]  SumNumOutMax=[]  DivideOutMin=[]  DivideOutMax=[]  UdiffTsProdOutMin=[]  UdiffTsProdOutMax=[]  NTsProdOutMin=[]  NTsProdOutMax=[]  UintegralTsProdOutMin=[]  UintegralTsProdOutMax=[]  UngainTsProdOutMin=[]  UngainTsProdOutMax=[]  ClampingZeroOutDataTypeStr=Inherit: Inherit via back propagation  ClampingZeroOutMin=[]  ClampingZeroOutMax=[]  FilterDenConstantOutDataTypeStr=Inherit: Inherit via back propagation  FilterDenConstantOutMin=[]  FilterDenConstantOutMax=[]  PCopyOutDataTypeStr=Inherit: Inherit via back propagation  PCopyOutMin=[]  PCopyOutMax=[]  NCopyOutDataTypeStr=Inherit: Inherit via back propagation  NCopyOutMin=[]  NCopyOutMax=[]  IntegratorContinuousStateAttributes=''  IntegratorStateMustResolveToSignalObject=off  IntegratorRTWStateStorageClass=Auto  FilterContinuousStateAttributes=''  FilterStateMustResolveToSignalObject=off  FilterRTWStateStorageClass=Auto  ParallelPVariant=ExternalParameters  IdealPVariant=Disabled  IVariant=ExternalParameters  DVariant=ExternalParameters  IntegratorVariant=Continuous  SatVariant=Enabled  AWVariant=Passthrough  PCopyVariant=Disabled  TRVariant=Disabled  FdbkBlocksVariant=Forward  IdealPFdbkVariant=Disabled  SatFdbkVariant=Disabled  DerivativeFilterVariant=ContFilter  NVariant=ExternalParameters  NCopyVariant=Disabled  FilterICVariant=InternalICsFilter  IntegratorICVariant=InternalICs  ExternalResetVariant=ExternalReset  TRSumVariant=Passthrough  SumFdbkVariant=Disabled  SumVariant=Sum_PID  TsampFilterVariant=InternalTs  TsampNgainVariant=Passthrough  TsampIntegralVariant=Passthrough  ExternalSaturationOutDataTypeStr=Inherit: Same as second input
  Actuator_controller_status_2 : Constant  Value=0
  Bus Selector1 : BusSelector  OutputSignals=Controller_P,Controller_I,Controller_D,Controller_N
  CloseLoop_disable_2 : Switch  Threshold=0.5  SaturateOnIntegerOverflow=off  InputSameDT=off
  Data Type Conversion : DataTypeConversion  OutDataTypeStr=double  SaturateOnIntegerOverflow=off  RndMeth=Floor
  Integrator reset determination : MATLAB Function  TreatAsAtomicUnit=on
  OR : Logic  Operator=OR  IconShape=distinctive  AllPortsSameDT=off  OutDataTypeStr=boolean
  Sum2 : Sum  Inputs=|-+  SaturateOnIntegerOverflow=on
  To Workspace1 : ToWorkspace  VariableName=error_act2  SampleTime=-1
  constant_ref_2 : Constant  Value=0
  enable_constant_ref_2 : Constant  Value=0
  ref_2 : Switch  Threshold=0.5  SaturateOnIntegerOverflow=off  InputSameDT=off
  reset_integrator_2 : Constant  Value=0
  Motor_current_2 : Outport
  wires:
  Bus Selector1/1 -> Actuator_PID_2/2  "<Controller_P>"
  Position/1 -> Sum2/1
  Actuator_PID_2/1 -> CloseLoop_disable_2/1
  Reference/1 -> ref_2/3
  [PID_Gains] -> Bus Selector1/1
  Bus Selector1/3 -> Actuator_PID_2/4  "<Controller_D>"
  Bus Selector1/4 -> Actuator_PID_2/5  "<Controller_N>"
  Init_current/1 -> CloseLoop_disable_2/3
  constant_ref_2/1 -> ref_2/1
  ref_2/1 -> Sum2/2
  enable_constant_ref_2/1 -> OR/2
  Sum2/1 -> To Workspace1/1, Actuator_PID_2/1
  Bus Selector1/2 -> Actuator_PID_2/3  "<Controller_I>"
  CloseLoop_disable_2/1 -> Motor_current_2/1
  Integrator reset determination/1(Integrator_reset_mode_2) -> Actuator_PID_2/6
  Actuator_controller_status_2/1 -> Integrator reset determination/1(closed_loop_disabled), CloseLoop_disable_2/2
  reset_integrator_2/1 -> Integrator reset determination/2(integrator_reset)
  OR/1 -> Data Type Conversion/1
  [enable_constant_ref_all] -> OR/1
  Data Type Conversion/1 -> ref_2/2

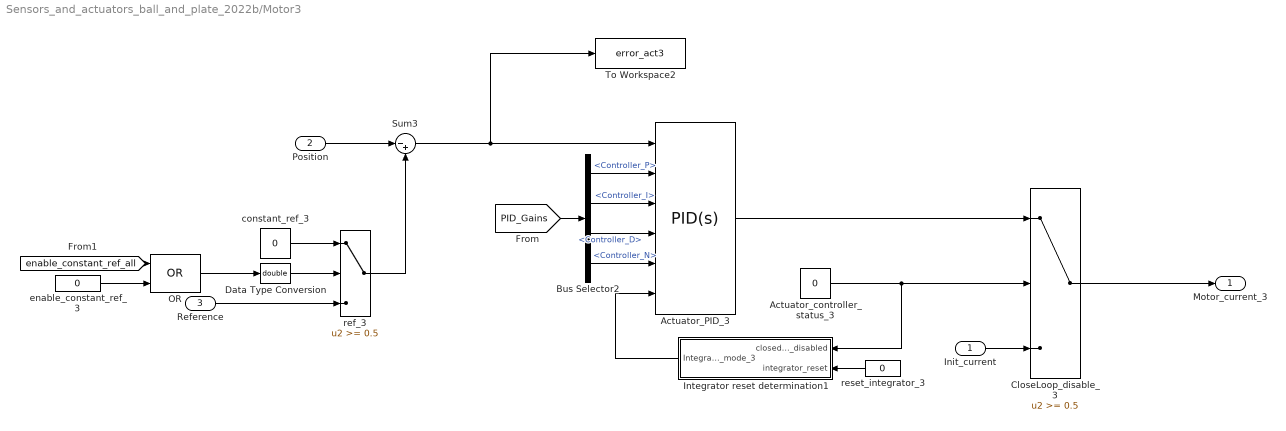
== system Sensors_and_actuators_ball_and_plate_2022b/Motor3 ==
  Init_current : Inport
  Position : Inport  Port=2
  Reference : Inport  Port=3
  Actuator_PID_3 : slpidlib/PID Controller  Controller=PID  Form=Parallel  TimeDomain=Continuous-time  UseExternalTs=off  SampleTime=-1  IntegratorMethod=Forward Euler  FilterMethod=Forward Euler  ControllerParametersSource=external  P=50  I=0  UseKiTs=off  D=0  N=100  UseFilter=on  TunerSelectOption=Transfer Function Based (PID Tuner App)  InitialConditionSource=internal  InitialConditionForIntegrator=0  InitialConditionForFilter=0  DifferentiatorICPrevScaledInput=0  ExternalReset=level  TrackingMode=off  Kt=1  LimitOutput=on  SatLimitsSource=internal  UpperSaturationLimit=3  LowerSaturationLimit=-3  LinearizeAsGain=on  AntiWindupMode=none  Kb=1  LimitIntegrator=off  UpperIntegratorSaturationLimit=inf  LowerIntegratorSaturationLimit=-inf  POutMin=[]  POutMax=[]  IOutMin=[]  IOutMax=[]  DOutMin=[]  DOutMax=[]  NOutMin=[]  NOutMax=[]  SumOutMin=[]  SumOutMax=[]  SaturationOutMin=[]  SaturationOutMax=[]  PParamMin=[]  PParamMax=[]  IParamMin=[]  IParamMax=[]  DParamMin=[]  DParamMax=[]  NParamMin=[]  NParamMax=[]  KbParamMin=[]  KbParamMax=[]  KtParamMin=[]  KtParamMax=[]  KbOutMin=[]  KbOutMax=[]  KtOutMin=[]  KtOutMax=[]  IntegratorOutMin=[]  IntegratorOutMax=[]  FilterOutMin=[]  FilterOutMax=[]  SumI1OutMin=[]  SumI1OutMax=[]  SumI2OutMin=[]  SumI2OutMax=[]  SumI3OutMin=[]  SumI3OutMax=[]  SumI4OutMin=[]  SumI4OutMax=[]  SumDOutMin=[]  SumDOutMax=[]  DifferentiatorOutMin=[]  DifferentiatorOutMax=[]  FilterDiffOutCoefMin=[]  FilterDiffOutCoefMax=[]  ReciprocalOutMin=[]  ReciprocalOutMax=[]  SumDenOutMin=[]  SumDenOutMax=[]  SumNumOutMin=[]  SumNumOutMax=[]  DivideOutMin=[]  DivideOutMax=[]  UdiffTsProdOutMin=[]  UdiffTsProdOutMax=[]  NTsProdOutMin=[]  NTsProdOutMax=[]  UintegralTsProdOutMin=[]  UintegralTsProdOutMax=[]  UngainTsProdOutMin=[]  UngainTsProdOutMax=[]  ClampingZeroOutDataTypeStr=Inherit: Inherit via back propagation  ClampingZeroOutMin=[]  ClampingZeroOutMax=[]  FilterDenConstantOutDataTypeStr=Inherit: Inherit via back propagation  FilterDenConstantOutMin=[]  FilterDenConstantOutMax=[]  PCopyOutDataTypeStr=Inherit: Inherit via back propagation  PCopyOutMin=[]  PCopyOutMax=[]  NCopyOutDataTypeStr=Inherit: Inherit via back propagation  NCopyOutMin=[]  NCopyOutMax=[]  IntegratorContinuousStateAttributes=''  IntegratorStateMustResolveToSignalObject=off  IntegratorRTWStateStorageClass=Auto  FilterContinuousStateAttributes=''  FilterStateMustResolveToSignalObject=off  FilterRTWStateStorageClass=Auto  ParallelPVariant=ExternalParameters  IdealPVariant=Disabled  IVariant=ExternalParameters  DVariant=ExternalParameters  IntegratorVariant=Continuous  SatVariant=Enabled  AWVariant=Passthrough  PCopyVariant=Disabled  TRVariant=Disabled  FdbkBlocksVariant=Forward  IdealPFdbkVariant=Disabled  SatFdbkVariant=Disabled  DerivativeFilterVariant=ContFilter  NVariant=ExternalParameters  NCopyVariant=Disabled  FilterICVariant=InternalICsFilter  IntegratorICVariant=InternalICs  ExternalResetVariant=ExternalReset  TRSumVariant=Passthrough  SumFdbkVariant=Disabled  SumVariant=Sum_PID  TsampFilterVariant=InternalTs  TsampNgainVariant=Passthrough  TsampIntegralVariant=Passthrough  ExternalSaturationOutDataTypeStr=Inherit: Same as second input
  Actuator_controller_status_3 : Constant  Value=0
  Bus Selector2 : BusSelector  OutputSignals=Controller_P,Controller_I,Controller_D,Controller_N
  CloseLoop_disable_3 : Switch  Threshold=0.5  SaturateOnIntegerOverflow=off  InputSameDT=off
  Data Type Conversion : DataTypeConversion  OutDataTypeStr=double  SaturateOnIntegerOverflow=off  RndMeth=Floor
  Integrator reset determination1 : MATLAB Function  TreatAsAtomicUnit=on
  OR : Logic  Operator=OR  IconShape=distinctive  AllPortsSameDT=off  OutDataTypeStr=boolean
  Sum3 : Sum  Inputs=|-+  SaturateOnIntegerOverflow=on
  To Workspace2 : ToWorkspace  VariableName=error_act3  SampleTime=-1
  constant_ref_3 : Constant  Value=0
  enable_constant_ref_3 : Constant  Value=0
  ref_3 : Switch  Threshold=0.5  SaturateOnIntegerOverflow=off  InputSameDT=off
  reset_integrator_3 : Constant  Value=0
  Motor_current_3 : Outport
  wires:
  Actuator_PID_3/1 -> CloseLoop_disable_3/1
  Reference/1 -> ref_3/3
  Bus Selector2/1 -> Actuator_PID_3/2  "<Controller_P>"
  [PID_Gains] -> Bus Selector2/1
  Sum3/1 -> To Workspace2/1, Actuator_PID_3/1
  ref_3/1 -> Sum3/2
  Bus Selector2/2 -> Actuator_PID_3/3  "<Controller_I>"
  Position/1 -> Sum3/1
  Bus Selector2/3 -> Actuator_PID_3/4  "<Controller_D>"
  Bus Selector2/4 -> Actuator_PID_3/5  "<Controller_N>"
  constant_ref_3/1 -> ref_3/1
  Init_current/1 -> CloseLoop_disable_3/3
  CloseLoop_disable_3/1 -> Motor_current_3/1
  Integrator reset determination1/1(Integrator_reset_mode_3) -> Actuator_PID_3/6
  Actuator_controller_status_3/1 -> CloseLoop_disable_3/2, Integrator reset determination1/1(closed_loop_disabled)
  reset_integrator_3/1 -> Integrator reset determination1/2(integrator_reset)
  [enable_constant_ref_all] -> OR/1
  enable_constant_ref_3/1 -> OR/2
  OR/1 -> Data Type Conversion/1
  Data Type Conversion/1 -> ref_3/2

== system Sensors_and_actuators_ball_and_plate_2022b/Outputs to Amplifier1 ==
  Motor current [A] : Inport
  Current2V : Gain  Gain=10/3  SaturateOnIntegerOverflow=on  OutDataTypeStr=Inherit: Same as input  ParamDataTypeStr=Inherit: Same as input
  DAC_CLASS1_BL1 : rti1202lib_dac_class1/DAC_CLASS1_BL1  DSProperties=struct('RTI',struct('Version',uint32(2),'BlockType',struct('isSLSource',uint8(0),'isSLSink',uint8(1),'isHWSource',uint8(0),'isHWSink',uint8(1),'isSetup',uint8(0),'isInline',uint8(1),'isNonInline',uint8(0),'isInterrupt',uint8(0),'isChannelwise',uint8(1)),'IOBoardType',{{'DS120X','STD','DACC1'}},'UnitType','DAC','Identifier','DAC','DialogType','ML','BlockSet','NONE','SlaveProcessor','NONE'))  RTIBlockInterface=struct('InputPortsActive',1,'InputPortsWidth',int32(1),'InputPortsDataType',{{'SS_DOUBLE'}},'InputPortsName',{{['DAC 1']}},'DialogFcn','rti120xstddacc1dacgui','InitLevel',3,'IconTransparency','on','BlockDisplay',{{['DAC CL1\nChannel: 1'],'center'}},'BlockName',struct('Token',{{'DAC_CLASS1_BL1'}}))  RTIBlockParameters=struct('ChannelNo',{{1,'OFF',[]}},'ChannelNumOf',{{1,'OFF',[]}},'InitialValue1',{{'0','OFF',[-10 10]}},'InitialValue2',{{'0','OFF',[-10 10]}},'InitialValue3',{{'0','OFF',[-10 10]}},'InitialValue4',{{'0','OFF',[-10 10]}},'InitialValue5',{{'0','OFF',[-10 10]}},'InitialValue6',{{'0','OFF',[-10 10]}},'InitialValue7',{{'0','OFF',[-10 10]}},'InitialValue8',{{'0','OFF',[-10 10]}},'InitialValue9',{{'0','OFF',[-10 10]}},'InitialValue10',{{'0','OFF',[-10 10]}},'InitialValue11',{{'0','OFF',[-10 10]}},'InitialValue12',{{'0','OFF',[-10 10]}},'InitialValue13',{{'0','OFF',[-10 10]}},'InitialValue14',{{'0','OFF',[-10 10]}},'InitialValue15',{{'0','OFF',[-10 10]}},'InitialValue16',{{'0','OFF',[-10 10]}},'OutputMode',{{ones(1,16),'OFF',[1 2]}},'TermValue1',{{'0','OFF',[-10 10]}},'TermValue2',{{'0','OFF',[-10 10]}},'TermValue3',{{'0','OFF',[-10 10]}},'TermValue4',{{'0','OFF',[-10 10]}},'TermValue5',{{'0','OFF',[-10 10]}},'TermValue6',{{'0','OFF',[-10 10]}},'TermValue7',{{'0','OFF',[-10 10]}},'TermValue8',{{'0','OFF',[-10 10]}},'TermValue9',{{'0','OFF',[-10 10]}},'TermValue10',{{'0','OFF',[-10 10]}},'TermValue11',{{'0','OFF',[-10 10]}},'TermValue12',{{'0','OFF',[-10 10]}},'TermValue13',{{'0','OFF',[-10 10]}},'TermValue14',{{'0','OFF',[-10 10]}},'TermValue15',{{'0','OFF',[-10 10]}},'TermValue16',{{'0','OFF',[-10 10]}},'EnableTermMode',{{0,'OFF',[0 1]}},'TLCFileName',{{'rti120xdac_c1_dac','OFF',[]}},'InitialValueBuildCheck1',{{1,'OFF',[]}},'InitialValueBuildCheck2',{{0,'OFF',[]}},'InitialValueBuildCheck3',{{0,'OFF',[]}},'InitialValueBuildCheck4',{{0,'OFF',[]}},'InitialValueBuildCheck5',{{0,'OFF',[]}},'InitialValueBuildCheck6',{{0,'OFF',[]}},'InitialValueBuildCheck7',{{0,'OFF',[]}},'InitialValueBuildCheck8',{{0,'OFF',[]}},'InitialValueBuildCheck9',{{0,'OFF',[]}},'InitialValueBuildCheck10',{{0,'OFF',[]}},'InitialValueBuildCheck11',{{0,'OFF',[]}},'InitialValueBuildCheck12',{{0,'OFF',[]}},'InitialValueBuildCheck13',{{0,'OFF',[]}},'InitialValueBuildCheck14',{{0,'OFF',[]}},'InitialValueBuildCheck15',{{0,'OFF',[]}},'InitialValueBuildCheck16',{{0,'OFF',[]}},'TermValueBuildCheck1',{{0,'OFF',[]}},'TermValueBuildCheck2',{{0,'OFF',[]}},'TermValueBuildCheck3',{{0,'OFF',[]}},'TermValueBuildCheck4',{{0,'OFF',[]}},'TermValueBuildCheck5',{{0,'OFF',[]}},'TermValueBuildCheck6',{{0,'OFF',[]}},'TermValueBuildCheck7',{{0,'OFF',[]}},'TermValueBuildCheck8',{{0,'OFF',[]}},'TermValueBuildCheck9',{{0,'OFF',[]}},'TermValueBuildCheck10',{{0,'OFF',[]}},'TermValueBuildCheck11',{{0,'OFF',[]}},'TermValueBuildCheck12',{{0,'OFF',[]}},'TermValueBuildCheck13',{{0,'OFF',[]}},'TermValueBuildCheck14',{{0,'OFF',[]}},'TermValueBuildCheck15',{{0,'OFF',[]}},'TermValueBuildCheck16',{{0,'OFF',[]}})  RTISFcnParameters=struct('ChannelNo','int16','ChannelNumOf','int16','InitialValue1','double','InitialValue2','double','InitialValue3','double','InitialValue4','double','InitialValue5','double','InitialValue6','double','InitialValue7','double','InitialValue8','double','InitialValue9','double','InitialValue10','double','InitialValue11','double','InitialValue12','double','InitialValue13','double','InitialValue14','double','InitialValue15','double','InitialValue16','double','OutputMode','int16','TermValue1','double','TermValue2','double','TermValue3','double','TermValue4','double','TermValue5','double','TermValue6','double','TermValue7','double','TermValue8','double','TermValue9','double','TermValue10','double','TermValue11','double','TermValue12','double','TermValue13','double','TermValue14','double','TermValue15','double','TermValue16','double','EnableTermMode','int16','TLCFileName','char')  RTIBlockParaDefault=struct('ChannelNo',1,'ChannelNumOf',1,'InitialValue1',0,'InitialValue2',0,'InitialValue3',0,'InitialValue4',0,'InitialValue5',0,'InitialValue6',0,'InitialValue7',0,'InitialValue8',0,'InitialValue9',0,'InitialValue10',0,'InitialValue11',0,'InitialValue12',0,'InitialValue13',0,'InitialValue14',0,'InitialValue15',0,'InitialValue16',0,'OutputMode',ones(1,16),'TermValue1',0,'TermValue2',0,'TermValue3',0,'TermValue4',0,'TermValue5',0,'TermValue6',0,'TermValue7',0,'TermValue8',0,'TermValue9',0,'TermValue10',0,'TermValue11',0,'TermValue12',0,'TermValue13',0,'TermValue14',0,'TermValue15',0,'TermValue16',0,'EnableTermMode',0,'TLCFileName','rti120xdac_c1_dac','InitialValueBuildCheck1',0,'InitialValueBuildCheck2',0,'InitialValueBuildCheck3',0,'InitialValueBuildCheck4',0,'InitialValueBuildCheck5',0,'InitialValueBuildCheck6',0,'InitialValueBuildCheck7',0,'InitialValueBuildCheck8',0,'InitialValueBuildCheck9',0,'InitialValueBuildCheck10',0,'InitialValueBuildCheck11',0,'InitialValueBuildCheck12',0,'InitialValueBuildCheck13',0,'InitialValueBuildCheck14',0,'InitialValueBuildCheck15',0,'InitialValueBuildCheck16',0,'TermValueBuildCheck1',0,'TermValueBuildCheck2',0,'TermValueBuildCheck3',0,'TermValueBuildCheck4',0,'TermValueBuildCheck5',0,'TermValueBuildCheck6',0,'TermValueBuildCheck7',0,'TermValueBuildCheck8',0,'TermValueBuildCheck9',0,'TermValueBuildCheck10',0,'TermValueBuildCheck11',0,'TermValueBuildCheck12',0,'TermValueBuildCheck13',0,'TermValueBuildCheck14',0,'TermValueBuildCheck15',0,'TermValueBuildCheck16',0)
  DSPscale : Gain  Gain=1/10  SaturateOnIntegerOverflow=on  OutDataTypeStr=Inherit: Same as input  ParamDataTypeStr=Inherit: Same as input
  MATLAB Function : MATLAB Function  TreatAsAtomicUnit=on
  Saturation : Saturate  UpperLimit=3  LowerLimit=-3
  saturationReached1 : Outport
  wires:
  Saturation/1 -> Current2V/1
  Current2V/1 -> DSPscale/1
  DSPscale/1 -> DAC_CLASS1_BL1/1
  Motor current [A]/1 -> MATLAB Function/1(current), Saturation/1
  MATLAB Function/1(saturation) -> saturationReached1/1
